simulink model "yawangleacc"  (R2020a)
settings: Solver=VariableStepAuto  StartTime=0.0  StopTime=10.0  RelTol=1e-3
undefined symbols (not defined in the file): Ixx, Iyy, Izz
settings Model: Creator=Muni Kumar  LastModifiedBy=Muni Kumar

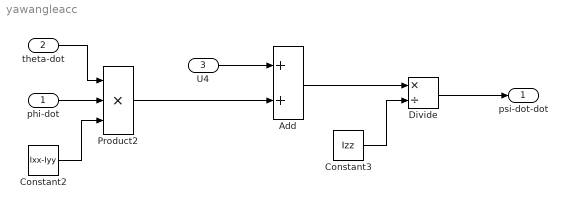
== system yawangleacc ==
  phi-dot : Inport
  theta-dot : Inport  Port=2
  U4 : Inport  Port=3
  Add : Sum
  Constant2 : Constant  Value=Ixx-Iyy
  Constant3 : Constant  Value=Izz
  Divide : Product  Inputs=*/
  Product2 : Product  Inputs=3
  psi-dot-dot : Outport
  wires:
  theta-dot/1 -> Product2/1
  Constant2/1 -> Product2/3
  Product2/1 -> Add/2
  phi-dot/1 -> Product2/2
  U4/1 -> Add/1
  Add/1 -> Divide/1
  Constant3/1 -> Divide/2
  Divide/1 -> psi-dot-dot/1
